simulink model "fuzzy_attack"  (R2021a)
settings: Solver=VariableStepAuto  StartTime=0.0  StopTime=10.0  RelTol=1e-3
values from neighbouring files (symbols this model uses):
  fuzzy_max_vs = 255/3.6    (= 70.8333333333)    [attack_setUp.m]
  fuzzy_min_vs = 0    [attack_setUp.m]
  probability = 2^(-4)    (= 0.0625)    [attack_setUp.m]
  seed_probability = 1    [attack_setUp.m]
settings Model: Creator=uidk9388  LastModifiedBy=uidk9388

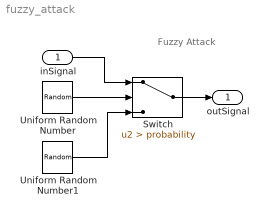
== system fuzzy_attack ==
  note: Fuzzy Attack
  inSignal : Inport
  Switch : Switch  Criteria=u2 > Threshold  Threshold=probability
  Uniform Random Number : UniformRandomNumber  Minimum=0  Seed=seed_probability  SampleTime=0.1
  Uniform Random Number1 : UniformRandomNumber  Minimum=fuzzy_min_vs  Maximum=fuzzy_max_vs  SampleTime=0.1
  outSignal : Outport
  wires:
  Uniform Random Number/1 -> Switch/2
  Uniform Random Number1/1 -> Switch/3
  inSignal/1 -> Switch/1
  Switch/1 -> outSignal/1
